simulink model "sampleModel1880_4_sub"  (R2023a)
settings: Solver=VariableStepAuto  StartTime=0.0  StopTime=10.0  RelTol=1e-3
libraries: hdlsllib x5, simulink x2
settings Model: Creator=user1  LastModifiedBy=user1
settings OptimizationCC: BlockReduction=off  ConditionallyExecuteInputs=off

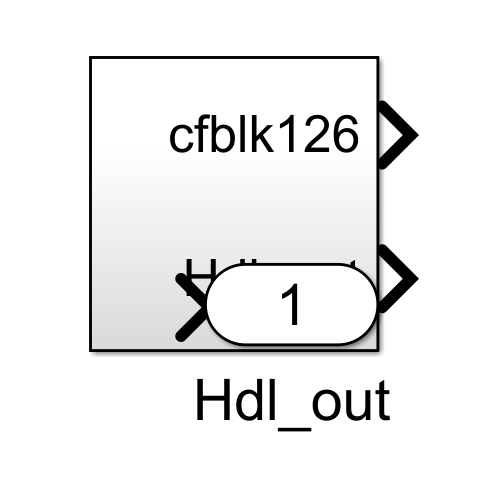
[thumbnail: Simulink's stored preview of the top-level diagram]
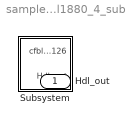
== system sampleModel1880_4_sub ==
  Subsystem : Subsystem
  Hdl_out : Outport  OutDataTypeStr=uint8

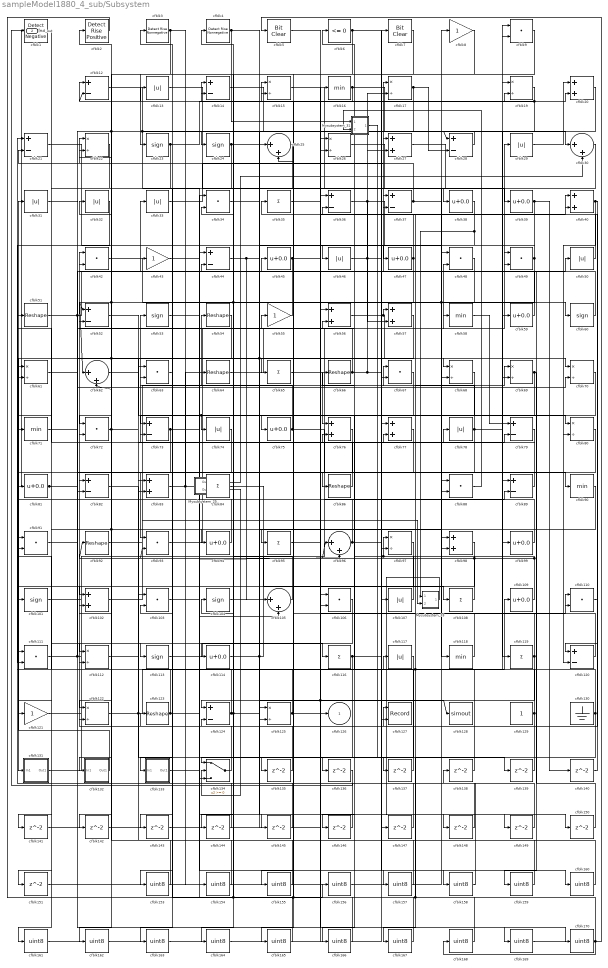
== system sampleModel1880_4_sub/Subsystem ==
  Mysubsystem_25 : Subsystem  TreatAsAtomicUnit=on  RTWFcnName=Mysubsystem_25
      settings: RTWFcnNameOpts=User specified  RTWFileNameOpts=Use function name
  Mysubsystem_31 : Subsystem  TreatAsAtomicUnit=on  RTWFcnName=Mysubsystem_31
      settings: RTWFcnNameOpts=User specified  RTWFileNameOpts=Use function name
  Mysubsystem_33 : Subsystem  TreatAsAtomicUnit=on  RTWFcnName=Mysubsystem_33
      settings: RTWFcnNameOpts=User specified  RTWFileNameOpts=Use function name
  cfblk1 : hdlsllib/Logic and Bit Operations/Detect Fall Negative  vinit=0  OutDataTypeStr=uint8
  cfblk{23..24,53,60,101,104,113} (7 alike) : Signum
  cfblk{20,27,40,56..57,76..77,83,98,102} (10 alike) : Sum  OutDataTypeStr=uint8
  cfblk{9,34,42,48..49,63,67,72,88,91,93,103,106,110..111} (15 alike) : DotProduct  OutDataTypeStr=uint8
  cfblk{25,30,62,96,105} (5 alike) : Sum  Inputs=|++  OutDataTypeStr=uint8
  cfblk{13,29,31..33,46,50,74,78,107,117} (11 alike) : Abs  OutDataTypeStr=uint8  SaturateOnIntegerOverflow=off
  cfblk{35,65,84,95,108,116,119} (7 alike) : Sum  Inputs=+  OutDataTypeStr=uint8
  cfblk{38..39,45,47,59,75,81,94,99,109,114} (11 alike) : Bias  Bias=0.0  SaturateOnIntegerOverflow=off
  cfblk{15,17,19,22,26,61,68..70,80,97,112,122,125} (14 alike) : Product  Inputs=*/  OutDataTypeStr=uint8  RndMeth=Zero  SaturateOnIntegerOverflow=on
  cfblk{16,58,71,90,118} (5 alike) : MinMax  OutDataTypeStr=uint8
  cfblk{12,14,21,28,36..37,44,52,73,79,82,89,120,124} (14 alike) : Sum  Inputs=+-  OutDataTypeStr=uint8
  cfblk{8,43,55,121} (4 alike) : Gain  OutDataTypeStr=uint8
  cfblk{51,54,64,66,86,92,123} (7 alike) : Reshape
  cfblk127 : Record  FileSettingsInternal="{\"entries\":[{\"content\":{\"excelSettings\":{\"content\":{},\"type\":\"Streamout.ExcelSettings\"}},\"type\":\"Streamout.FileSettingStorage\",\"uuid\":\"\"}],\"packageUris\":[\"http:\\/\\/schema.mathworks.com\\/mf0\\/streamout_blocks\\/R2020a\"],\"version\":\"1.0\"}"  Layout=[1 1]  SignalsInternal="{\"entries\":[{\"content\":{\"signals\":[{\"content\":{\"blockPath\":[],\"dimensions\":[1],\"domain\":\"\",\"lineColor\":\"#a2142f\",\"plots\":[1],\"port\":1,\"signalID\":46700,\"signalName\":\"cfblk110\"},\"type\":\"RecordBlkView.Signal\",\"uuid\":\"\"},{\"content\":{\"blockPath\":[],\"dimensions\":[1],\"domain\":\"\",\"lineColor\":\"#139fff\",\"plots\":[1],\"port\":2,\"signalID\":46703,\"signalName\":\"cfblk4\"},\"type\":\"RecordBlkView.Signal\",\"uuid\":\"\"}]},\"type\":\"RecordBlkView.InputSignals\",\"uuid\":\"\"}],\"packageUris\":[\"http:\\/\\/schema.mathworks.com\\/mf0\\/streamout_blocks\\/R2020a\"],\"version\":\"1.0\"}"  VisualizationBindings="{\"xyplotplugin\":{\"info\":[{\"series\":[{\"bindingParametersList\":[{\"parameter\":\"X-Axis\",\"signalID\":46700,\"signalName\":\"cfblk110\"},{\"parameter\":\"Y-Axis\",\"signalID\":46703,\"signalName\":\"cfblk4\"}],\"seriesID\":18294}],\"subplotID\":1}]}}"  CompatibilityTag=XY  st=-1
  cfblk128 : ToWorkspace  VariableName=simout  SaveFormat=Timeseries  SampleTime=-1
  cfblk129 : Constant  OutDataTypeStr=uint8  SampleTime=-1
  cfblk130 : Ground
  cfblk131 : Subsystem
      settings: LibrarySourceBlock=|
      | hdlsllib/Ports &
      | Subsystems/Subsystem
  cfblk132 : Subsystem
      settings: LibrarySourceBlock=|
      | hdlsllib/Ports &
      | Subsystems/Subsystem
  cfblk133 : Subsystem
      settings: LibrarySourceBlock=|
      | hdlsllib/Ports &
      | Subsystems/Subsystem
  cfblk134 : Switch  OutDataTypeStr=uint8  SaturateOnIntegerOverflow=off  InputSameDT=off
  cfblk{135..151} (17 alike) : Delay  SampleTime=1
  cfblk{153..170} (18 alike) : DataTypeConversion  OutDataTypeStr=uint8  SaturateOnIntegerOverflow=off  RndMeth=Floor
  cfblk2 : hdlsllib/Logic and Bit Operations/Detect Rise Positive  vinit=0  OutDataTypeStr=uint8
  cfblk3 : hdlsllib/Logic and Bit Operations/Detect Rise Nonnegative  vinit=0  OutDataTypeStr=uint8
  cfblk4 : hdlsllib/Logic and Bit Operations/Detect Rise Nonnegative  vinit=0  OutDataTypeStr=uint8
  cfblk5 : simulink/Logic and Bit Operations/Bit Clear  iBit=0
      settings: LibrarySourceBlock=|
      | hdlsllib/Logic and Bit
      | Operations/Bit Clear
  cfblk6 : hdlsllib/Logic and Bit Operations/Compare To Zero  relop=<=  OutDataTypeStr=uint8
  cfblk7 : simulink/Logic and Bit Operations/Bit Clear  iBit=0
      settings: LibrarySourceBlock=|
      | hdlsllib/Logic and Bit
      | Operations/Bit Clear
  cfblk126 : Outport  OutDataTypeStr=uint8  VectorParamsAs1DForOutWhenUnconnected=off
  Hdl_out : Outport  Port=2  OutDataTypeStr=uint8
  wires:
  cfblk134/1 -> cfblk42/1
  cfblk14/1 -> cfblk30/1
  cfblk109/1 -> cfblk52/2, cfblk92/1
  cfblk84/1 -> cfblk108/1
  cfblk89/1 -> cfblk53/1
  cfblk13/1 -> cfblk38/1
  cfblk58/1 -> cfblk79/1
  cfblk3/1 -> cfblk154/1, cfblk23/1
  cfblk101/1 -> cfblk29/1
  cfblk132/1(Out1) -> cfblk31/1
  cfblk67/1 -> cfblk75/1
  cfblk60/1 -> cfblk12/1
  cfblk57/1 -> cfblk131/1(In1)
  cfblk21/1 -> cfblk98/1
  cfblk42/1 -> cfblk89/1
  cfblk119/1 -> cfblk144/1, cfblk14/2
  cfblk118/1 -> cfblk55/1
  cfblk22/1 -> cfblk71/1
  cfblk65/1 -> cfblk76/1
  cfblk102/1 -> cfblk54/1
  cfblk15/1 -> cfblk39/1
  cfblk124/1 -> cfblk109/1, cfblk150/1, cfblk34/2
  cfblk47/1 -> cfblk6/1, cfblk114/1, cfblk62/1
  cfblk69/1 -> cfblk159/1, cfblk94/1
  cfblk50/1 -> cfblk25/2
  cfblk38/1 -> cfblk46/1, Mysubsystem_33/1(In1)
  cfblk105/1 -> cfblk4/1
  cfblk51/1 -> cfblk67/2, cfblk33/1
  cfblk64/1 -> cfblk49/1
  cfblk59/1 -> cfblk17/1
  cfblk121/1 -> cfblk9/1
  cfblk44/1 -> cfblk105/1, cfblk125/1
  cfblk76/1 -> cfblk93/1
  cfblk86/1 -> cfblk51/1
  cfblk93/1 -> cfblk48/2
  cfblk131/1(Out1) -> cfblk89/2
  cfblk49/1 -> cfblk124/1, cfblk47/1
  cfblk77/1 -> cfblk166/1
  cfblk36/1 -> cfblk57/2, cfblk118/1
  cfblk112/1 -> cfblk83/2
  cfblk68/1 -> cfblk86/1
  cfblk61/1 -> cfblk50/1
  cfblk80/1 -> cfblk95/1
  cfblk23/1 -> cfblk20/2, cfblk72/1
  cfblk25/1 -> cfblk73/1
  cfblk73/1 -> cfblk105/2, cfblk91/1
  cfblk35/1 -> cfblk126/1
  cfblk48/1 -> cfblk88/2, cfblk113/1
  cfblk130/1 -> cfblk167/1, cfblk13/1
  cfblk123/1 -> cfblk69/1, cfblk72/2
  cfblk116/1 -> cfblk164/1, cfblk110/2
  cfblk122/1 -> cfblk79/2, cfblk9/2
  cfblk107/1 -> cfblk81/1, cfblk97/1
  cfblk31/1 -> cfblk90/1
  cfblk29/1 -> cfblk20/1
  cfblk9/1 -> cfblk134/1
  cfblk17/1 -> cfblk28/2, cfblk82/2, cfblk122/1
  cfblk8/1 -> cfblk97/2
  cfblk113/1 -> cfblk116/1
  cfblk4/1 -> cfblk69/2, cfblk127/2, Mysubsystem_31/1(In1)
  cfblk111/1 -> cfblk58/1, cfblk26/1
  cfblk114/1 -> cfblk78/1, cfblk8/1
  cfblk125/1 -> cfblk82/1, cfblk128/1, cfblk110/1
  cfblk83/1 -> cfblk64/1, cfblk96/2, cfblk16/1
  cfblk19/1 -> cfblk142/1, cfblk12/2
  cfblk110/1 -> cfblk127/1
  cfblk72/1 -> cfblk80/1, cfblk132/1(In1)
  cfblk97/1 -> cfblk121/1
  cfblk32/1 -> cfblk111/2
  cfblk37/1 -> cfblk21/2, cfblk70/1
  cfblk52/1 -> cfblk80/2, cfblk74/1
  cfblk98/1 -> cfblk133/1(In1), cfblk93/2
  cfblk33/1 -> cfblk27/1
  cfblk91/1 -> cfblk56/2
  cfblk5/1 -> cfblk170/1
  cfblk1/1 -> cfblk101/1
  cfblk27/1 -> cfblk99/1
  cfblk94/1 -> cfblk42/2
  cfblk7/1 -> cfblk165/1
  cfblk129/1 -> cfblk122/2, cfblk66/1, cfblk37/1
  cfblk6/1 -> cfblk162/1, cfblk148/1
  cfblk24/1 -> cfblk134/3, cfblk26/2
  cfblk45/1 -> cfblk44/2, cfblk40/1
  cfblk56/1 -> cfblk68/1, cfblk57/1
  cfblk39/1 -> cfblk140/1, cfblk125/2
  cfblk81/1 -> Hdl_out/1, cfblk70/2
  cfblk54/1 -> cfblk62/2, cfblk61/2
  cfblk120/1 -> cfblk22/1
  cfblk34/1 -> cfblk98/2
  cfblk46/1 -> cfblk27/2, cfblk60/1
  cfblk108/1 -> cfblk14/1, cfblk96/1
  cfblk78/1 -> cfblk146/1, cfblk37/2, cfblk19/1
  cfblk28/1 -> cfblk24/1
  cfblk62/1 -> cfblk65/1
  cfblk99/1 -> cfblk36/2
  cfblk12/1 -> cfblk28/1, cfblk84/1
  cfblk96/1 -> cfblk160/1, cfblk15/1
  cfblk75/1 -> cfblk43/1, cfblk119/1
  cfblk16/1 -> cfblk15/2, cfblk59/1
  cfblk20/1 -> cfblk52/1, cfblk102/1
  cfblk66/1 -> cfblk3/1, cfblk17/2, cfblk19/2
  cfblk133/1(Out1) -> cfblk67/1
  cfblk79/1 -> cfblk76/2
  cfblk55/1 -> cfblk45/1
  cfblk26/1 -> cfblk88/1
  cfblk40/1 -> cfblk120/2, cfblk120/1
  cfblk90/1 -> cfblk151/1, cfblk112/1
  cfblk53/1 -> cfblk135/1
  cfblk135/1 -> cfblk73/2
  cfblk136/1 -> cfblk1/1
  cfblk82/1 -> cfblk137/1
  cfblk137/1 -> cfblk91/2
  cfblk138/1 -> cfblk111/1
  cfblk104/1 -> cfblk139/1
  cfblk139/1 -> cfblk48/1
  cfblk140/1 -> cfblk40/2
  cfblk30/1 -> cfblk141/1
  cfblk141/1 -> cfblk25/1
  cfblk142/1 -> cfblk112/2
  cfblk70/1 -> cfblk143/1
  cfblk143/1 -> cfblk36/1
  cfblk144/1 -> cfblk21/1
  cfblk43/1 -> cfblk145/1
  cfblk145/1 -> cfblk83/1
  cfblk146/1 -> cfblk22/2
  cfblk147/1 -> cfblk61/1
  cfblk148/1 -> cfblk102/2
  cfblk149/1 -> cfblk56/1
  cfblk150/1 -> cfblk49/2
  cfblk151/1 -> cfblk68/2
  cfblk63/1 -> cfblk153/1
  cfblk153/1 -> cfblk32/1
  cfblk154/1 -> cfblk63/1
  cfblk117/1 -> cfblk155/1
  cfblk155/1 -> cfblk63/2
  cfblk2/1 -> cfblk156/1
  cfblk156/1 -> cfblk107/1
  cfblk95/1 -> cfblk157/1
  cfblk157/1 -> cfblk2/1
  cfblk103/1 -> cfblk158/1
  cfblk158/1 -> cfblk138/1
  cfblk159/1 -> cfblk103/1
  cfblk160/1 -> cfblk103/2
  cfblk106/1 -> cfblk161/1
  cfblk161/1 -> cfblk147/1
  cfblk162/1 -> cfblk106/1
  cfblk74/1 -> cfblk163/1
  cfblk163/1 -> cfblk106/2
  cfblk164/1 -> cfblk7/1
  cfblk165/1 -> cfblk44/1, cfblk104/1
  cfblk166/1 -> cfblk35/1, cfblk123/1, cfblk124/2
  cfblk167/1 -> cfblk77/1
  cfblk168/1 -> cfblk77/2
  cfblk71/1 -> cfblk169/1
  cfblk169/1 -> cfblk5/1
  cfblk170/1 -> cfblk168/1, cfblk117/1, cfblk34/1
  Mysubsystem_25/1(Out1) -> cfblk30/2
  Mysubsystem_25/2(Out2) -> cfblk134/2
  cfblk88/1 -> Mysubsystem_31/2(In2)
  Mysubsystem_31/1(Out1) -> cfblk136/1
  cfblk92/1 -> Mysubsystem_33/2(In2)
  Mysubsystem_33/1(Out1) -> cfblk149/1

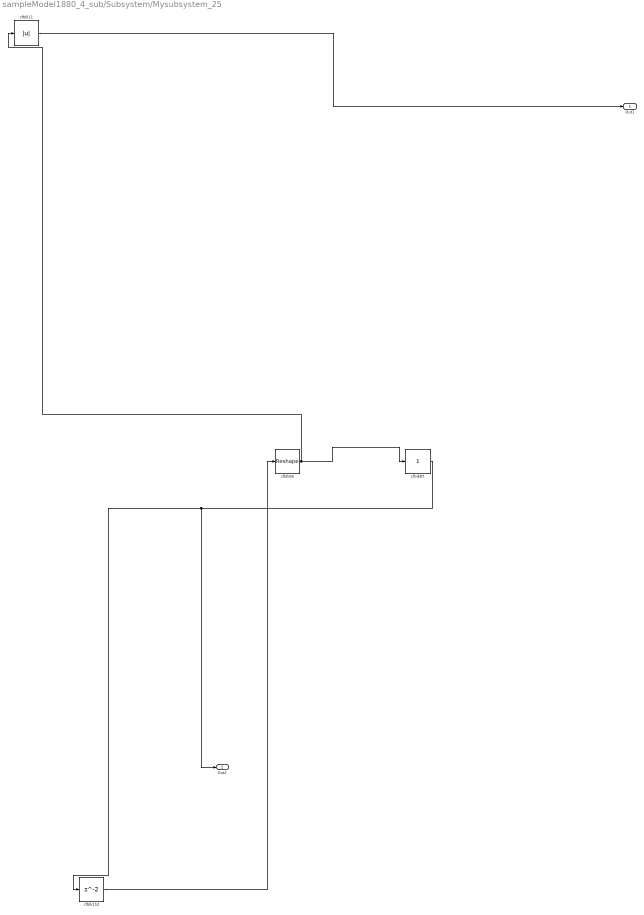
== system sampleModel1880_4_sub/Subsystem/Mysubsystem_25 ==
  cfblk11 : Abs  SaturateOnIntegerOverflow=off
  cfblk152 : Delay  SampleTime=1
  cfblk85 : Reshape
  cfblk87 : Sum  Inputs=+
  Out1 : Outport
  Out2 : Outport  Port=2
  wires:
  cfblk11/1 -> Out1/1
  cfblk85/1 -> cfblk11/1, cfblk87/1
  cfblk87/1 -> cfblk152/1, Out2/1
  cfblk152/1 -> cfblk85/1

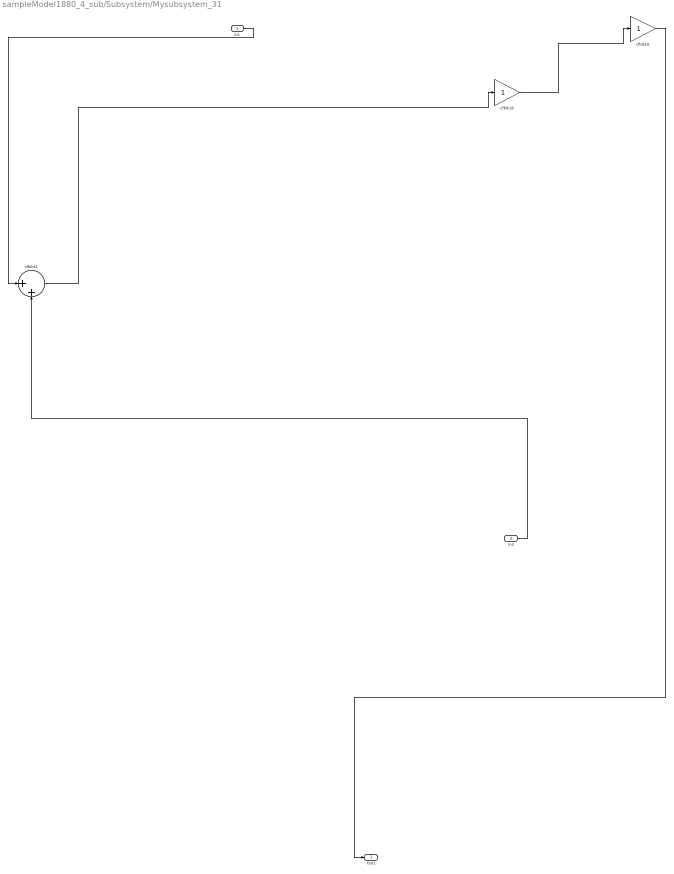
== system sampleModel1880_4_sub/Subsystem/Mysubsystem_31 ==
  In1 : Inport
  In2 : Inport  Port=2
  cfblk10 : Gain
  cfblk18 : Gain
  cfblk41 : Sum  Inputs=|++
  Out1 : Outport
  wires:
  cfblk10/1 -> Out1/1
  In1/1 -> cfblk41/1
  cfblk41/1 -> cfblk18/1
  In2/1 -> cfblk41/2
  cfblk18/1 -> cfblk10/1

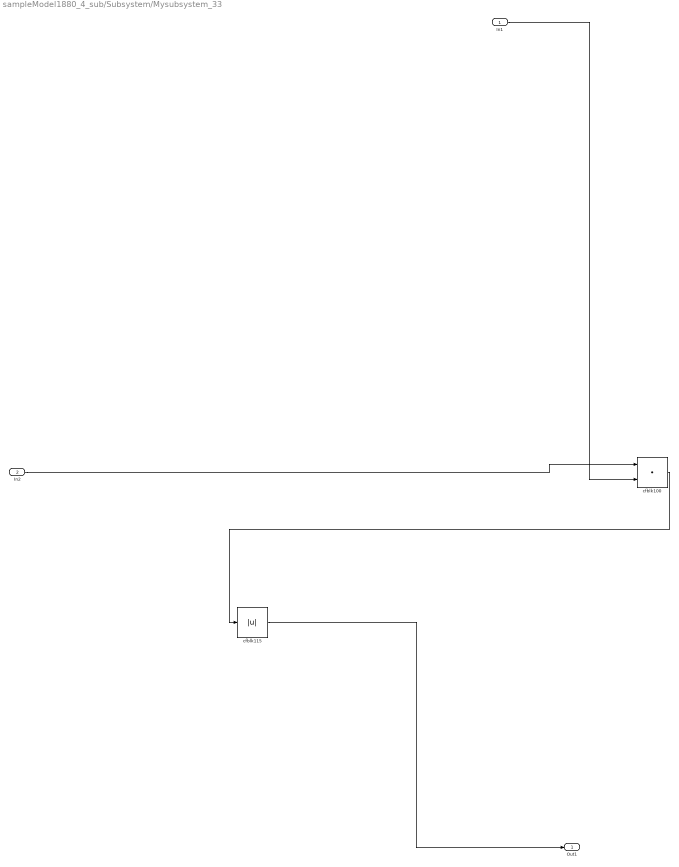
== system sampleModel1880_4_sub/Subsystem/Mysubsystem_33 ==
  In1 : Inport
  In2 : Inport  Port=2
  cfblk100 : DotProduct  OutDataTypeStr=Inherit: Inherit via internal rule
  cfblk115 : Abs  SaturateOnIntegerOverflow=off
  Out1 : Outport
  wires:
  In1/1 -> cfblk100/2
  In2/1 -> cfblk100/1
  cfblk115/1 -> Out1/1
  cfblk100/1 -> cfblk115/1

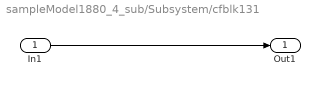
== system sampleModel1880_4_sub/Subsystem/cfblk131 ==
  In1 : Inport
  Out1 : Outport
  wires:
  In1/1 -> Out1/1

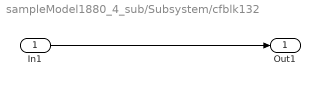
== system sampleModel1880_4_sub/Subsystem/cfblk132 ==
  In1 : Inport
  Out1 : Outport
  wires:
  In1/1 -> Out1/1

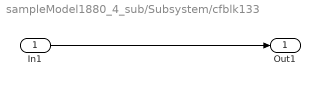
== system sampleModel1880_4_sub/Subsystem/cfblk133 ==
  In1 : Inport
  Out1 : Outport
  wires:
  In1/1 -> Out1/1
